simulink model "Examen_parte2"  (R2013a)
settings: Solver=ode45  StartTime=0.0  StopTime=10.0  RelTol=1e-3
settings Model: Creator=Miguel  LastModifiedBy=Miguel

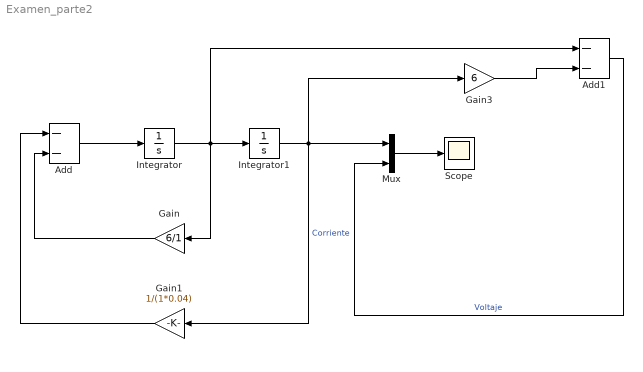
== system Examen_parte2 ==
  Add : Sum  Inputs=--
  Add1 : Sum  Inputs=--
  Gain : Gain  Gain=6/1
  Gain1 : Gain  Gain=1/(1*0.04)
  Gain3 : Gain  Gain=6
  Integrator : Integrator  InitialCondition=-1/1*(6*4-4)
  Integrator1 : Integrator  InitialCondition=4
  Mux : Mux  Inputs=2
  Scope : Scope
      settings: ShowLegends=on
  wires:
  Integrator/1 -> Gain/1, Add1/1, Integrator1/1
  Integrator1/1 -> Gain3/1, Gain1/1, Mux/1  "Corriente"
  Mux/1 -> Scope/1
  Add/1 -> Integrator/1
  Gain1/1 -> Add/1
  Gain/1 -> Add/2
  Gain3/1 -> Add1/2
  Add1/1 -> Mux/2  "Voltaje"
